simulink subsystem "Thruster_Solver_Subsystem"  (R2023a)
settings: Solver=VariableStepAuto  StartTime=0.0  StopTime=10.0  RelTol=1e-3

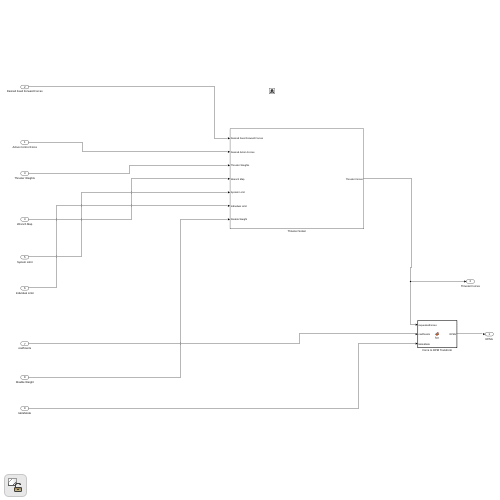
[thumbnail: Simulink's stored preview of the top-level diagram]
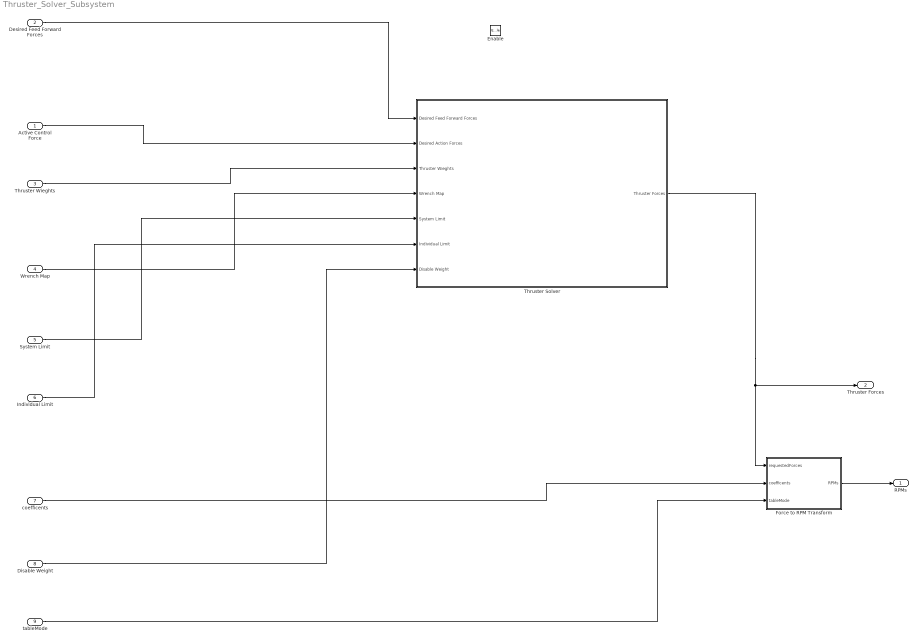
== system Thruster_Solver_Subsystem ==
  Active Control Force : Inport
  Desired Feed Forward Forces : Inport  Port=2
  Thruster Wieghts : Inport  Port=3
  Wrench Map : Inport  Port=4
  System Limit : Inport  Port=5
  Individual Limit : Inport  Port=6
  coefficents : Inport  Port=7
  Disable Weight : Inport  Port=8
  tableMode : Inport  Port=9
  Enable : EnablePort
  Force to RPM Transform : MATLAB Function  TreatAsAtomicUnit=on
  Thruster Solver : Subsystem
  RPMs : Outport
  Thruster Forces : Outport  Port=2
  wires:
  System Limit/1 -> Thruster Solver/5(System Limit)
  tableMode/1 -> Force to RPM Transform/3(tableMode)
  coefficents/1 -> Force to RPM Transform/2(coefficents)
  Thruster Wieghts/1 -> Thruster Solver/3(Thruster Wieghts)
  Thruster Solver/1(Thruster Forces) -> Force to RPM Transform/1(requestedForces), Thruster Forces/1
  Disable Weight/1 -> Thruster Solver/7(Disable Weight)
  Active Control Force/1 -> Thruster Solver/2(Desired Action Forces)
  Individual Limit/1 -> Thruster Solver/6(Individual Limit)
  Desired Feed Forward Forces/1 -> Thruster Solver/1(Desired Feed Forward Forces)
  Wrench Map/1 -> Thruster Solver/4(Wrench Map)
  Force to RPM Transform/1(RPMs) -> RPMs/1

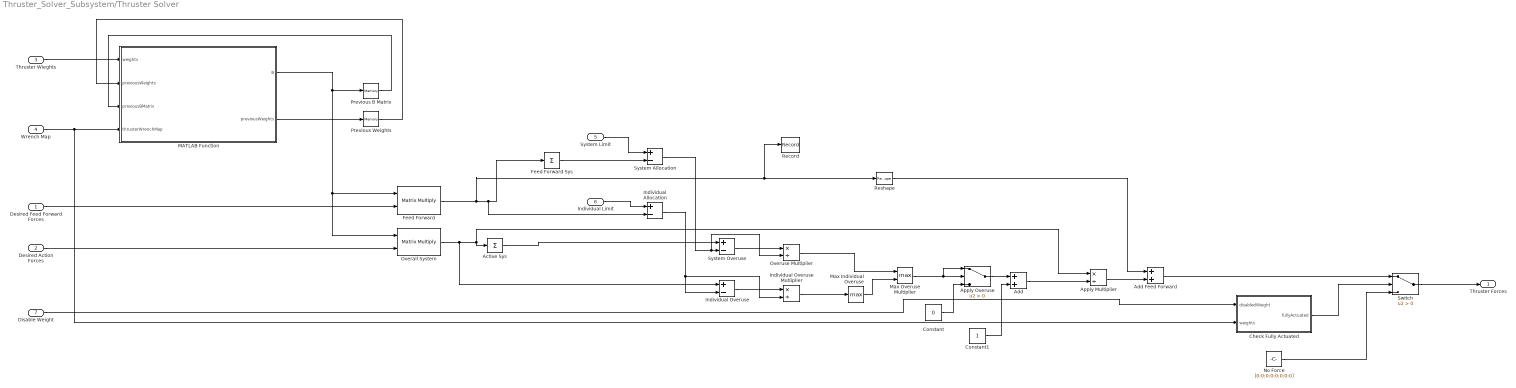
== system Thruster_Solver_Subsystem/Thruster Solver ==
  Desired Feed Forward Forces : Inport  PortDimensions=[6 1]
  Desired Action Forces : Inport  Port=2  PortDimensions=[6 1]
  Thruster Wieghts : Inport  Port=3  PortDimensions=[8 1]
  Wrench Map : Inport  Port=4
  System Limit : Inport  Port=5
  Individual Limit : Inport  Port=6
  Disable Weight : Inport  Port=7
  Active Sys : Sum  Inputs=+
  Add : Sum
  Add Feed Forward : Sum  AccumDataTypeStr=double
  Apply Multiplier : Product  Inputs=*/  OutDataTypeStr=double
  Apply Overuse : Switch  Criteria=u2 > Threshold  SaturateOnIntegerOverflow=off  InputSameDT=off
  Check Fully Actuated : MATLAB Function  TreatAsAtomicUnit=on
  Constant : Constant  Value=0
  Constant1 : Constant
  "Feed Forward " : Product  Multiplication=Matrix(*)
  Feed Forward Sys : Sum  Inputs=+
  Individual Allocation : Sum  Inputs=+-
  Individual Overuse : Sum  Inputs=+-
  Individual Overuse Mutliplier : Product  Inputs=*/
  MATLAB Function : MATLAB Function  TreatAsAtomicUnit=on
  Max Individual Overuse : MinMax  Function=max
  Max Overuse Multiplier : MinMax  Function=max  Inputs=2
  No Force : Constant  Value=[0;0;0;0;0;0;0;0]
  Overall System : Product  Multiplication=Matrix(*)
  Overuse Multiplier : Product  Inputs=*/
  Previous B Matrix : Memory  InitialCondition=[inf inf inf inf inf inf; inf inf inf inf inf inf; inf inf inf inf inf inf; inf inf inf inf inf inf; inf inf inf inf inf inf; inf inf inf inf inf inf; inf inf inf inf inf inf; inf inf inf inf inf inf]  InheritSampleTime=on
  Previous Weights : Memory  InitialCondition=[ inf inf inf inf inf inf inf inf]  InheritSampleTime=on
  Record : Record  FileSettingsInternal="{\"entries\":[{\"content\":{\"excelSettings\":{\"content\":{},\"type\":\"Streamout.ExcelSettings\"}},\"type\":\"Streamout.FileSettingStorage\",\"uuid\":\"\"}],\"packageUris\":[\"http:\\/\\/schema.mathworks.com\\/mf0\\/streamout_blocks\\/R2020a\"],\"version\":\"1.0\"}"  SignalsInternal="{\"entries\":[{\"content\":{\"signals\":[{\"content\":{\"blockPath\":[],\"dimensions\":[8,1],\"domain\":\"\",\"hasChildren\":true,\"lineColor\":\"#77ac30\",\"port\":1,\"signalID\":827,\"signalName\":\"Feed Forward \"},\"type\":\"RecordBlkView.Signal\",\"uuid\":\"\"},{\"content\":{\"blockPath\":[],\"channel\":[1,1],\"dimensions\":[8,1],\"domain\":\"\",\"lineColor\":\"#d95319\",\"parentID\":827,\"plots\":[1],\"port\":1,\"signalID\":828,\"signalName\":\"Feed Forwa ...(+1670 chars)"  VisualizationBindings="{\"sparklinesplugin\":{\"info\":[{\"bindingParametersList\":[],\"subplotID\":1}]}}"
  Reshape : Reshape  OutputDimensionality=Column vector (2-D)
  Switch : Switch  Criteria=u2 > Threshold  SaturateOnIntegerOverflow=off  InputSameDT=off
  System Allocation : Sum  Inputs=+-
  System Overuse : Sum  Inputs=+-
  Thruster Forces : Outport
  wires:
  Switch/1 -> Thruster Forces/1
  No Force/1 -> Switch/3
  Disable Weight/1 -> Check Fully Actuated/1(disabledWeight)
  Check Fully Actuated/1(fullyActuated) -> Switch/2
  Reshape/1 -> Add Feed Forward/1
  MATLAB Function/2(previousWeights) -> Previous Weights/1
  Individual Limit/1 -> Individual Allocation/1
  System Limit/1 -> System Allocation/1
  Previous Weights/1 -> MATLAB Function/2("previousWeights ")
  Thruster Wieghts/1 -> MATLAB Function/1(weights)
  Wrench Map/1 -> MATLAB Function/4(thrusterWrenchMap), Check Fully Actuated/2(weights)
  Previous B Matrix/1 -> MATLAB Function/3(previousBMatrix)
  MATLAB Function/1(B) -> Previous B Matrix/1, "Feed Forward "/1, Overall System/1
  Add Feed Forward/1 -> Switch/1
  Add/1 -> Apply Multiplier/2
  Apply Overuse/1 -> Add/1
  Individual Overuse Mutliplier/1 -> Max Individual Overuse/1
  Constant1/1 -> Add/2
  "Feed Forward "/1 -> Feed Forward Sys/1, Individual Allocation/2, Reshape/1, Record/1
  Desired Action Forces/1 -> Overall System/2
  System Allocation/1 -> System Overuse/2, Overuse Multiplier/2
  Max Individual Overuse/1 -> Max Overuse Multiplier/2
  Overuse Multiplier/1 -> Max Overuse Multiplier/1
  Apply Multiplier/1 -> Add Feed Forward/2
  Active Sys/1 -> System Overuse/1
  System Overuse/1 -> Overuse Multiplier/1
  Desired Feed Forward Forces/1 -> "Feed Forward "/2
  Max Overuse Multiplier/1 -> Apply Overuse/2, Apply Overuse/1
  Overall System/1 -> Active Sys/1, Apply Multiplier/1, Individual Overuse/1
  Individual Allocation/1 -> Individual Overuse/2, Individual Overuse Mutliplier/2
  Individual Overuse/1 -> Individual Overuse Mutliplier/1
  Feed Forward Sys/1 -> System Allocation/2
  Constant/1 -> Apply Overuse/3

== matlab function Thruster_Solver_Subsystem/Force to RPM Transform ==
function RPMs = fcn(requestedForces, coefficents, tableMode)

%the output array with rpm values
RPMs = zeros([8,1]);

if(tableMode)
   %evaluate each thruster -- discontinuos curve
    for i = 1:8
        requestedForce = requestedForces(i);
    
        if(requestedForce > .01)
            %positive curve
            RPMs(i) = 120 + sin(requestedForce/ 60 * pi) ^ (1/3) * 130;
            RPMs(i) = min(250, RPMs(i));
        elseif(requestedForce < -.01)
            %negative curve
            RPMs(i) = -120 - (abs(sin(requestedForce/ 60 * pi)) ^ (1/3)) * 130;
            RPMs(i) = max(-250, RPMs(i));  
        end
    end 

else

    %evaluate each thruster -- discontinuos curve
    for i = 1:8
        requestedForce = requestedForces(i);
        
        if(requestedForce > 0)
            %positive curve
            RPMs(i) = round(coefficents(1) + coefficents(2) * requestedForces(i) + coefficents(3) * tanh(requestedForces(i)) + requestedForces(i)^(1/4) * coefficents(4));
        else
            %negative curve
            RPMs(i) = round(coefficents(5) + coefficents(6) * requestedForces(i) + coefficents(7) * tanh(requestedForces(i)) + abs(requestedForces(i))^(1/4) * coefficents(8));
        end
    
    end

end

== matlab function Thruster_Solver_Subsystem/Thruster Solver/Check Fully Actuated ==
function fullyActuated = fcn(disabledWeight, weights)

enabled_thrusters = 0;

%count number of enabled thrusters
for i = 1:length(weights)
    if(weights(i) < disabledWeight)
        enabled_thrusters = enabled_thrusters + 1;
    end
end

%if enough thrusters to be fully actuated allow forces
if(enabled_thrusters >= 6)
    fullyActuated = 1;

    return
end

fullyActuated = 0;

== matlab function Thruster_Solver_Subsystem/Thruster Solver/MATLAB Function ==
function [B,previousWeights] = generateBMatrix(weights, previousWeights, previousBMatrix, thrusterWrenchMap)

    if(isequal(weights, previousWeights))
        %if the weights are the same, just send the previous B matrix
        B = previousBMatrix;
        return
    end

    %if new weights, calculate the a new b matrix
    weightsMatrix = diag(weights);
    B = inv(weightsMatrix) * (thrusterWrenchMap) * inv((transpose(thrusterWrenchMap) * inv(weightsMatrix) * (thrusterWrenchMap)))
    previousWeights = weights;
end
